simulink model "eVTOL_PX4_2023b"  (R2024b)
settings: Solver=ode4  StartTime=0  StopTime=inf  FixedStep=0.01  RelTol=1e-3
values from neighbouring files (symbols this model uses):
  aDl =     [initdata.mat]
  aDr =     [initdata.mat]
  aDyn =     [initdata.mat]
  Airport = init_airport('PHNL')    [initdata_HIL_eVTOL.m]
  aLat =     [initdata.mat]
  aLon =     [initdata.mat]
  D = Prop.D    [EOM_dt_MC.m]    (also in EOM_get_alf_dt_de_prop_evtol.m = CD * QS)
  dt0 = X(2)    [EOM_get_alf_dt_de_prop_evtol.m]    (also in initdata.mat = 0.258252593971; initdata_HIL_eVTOL.m = EOM_dt_MC)
  EAS0 = TAS0 / EAS2TAS    [initdata_HIL_eVTOL.m]
  FCS = init_FCS    [initdata_HIL_eVTOL.m]
  General = init_layoutdata    [EOM_dt_MC.m]    (also in build_optimized_CA.m; initdata.mat = ; initdata_HIL_eVTOL.m)
  h0 = Con(1)    [EOM_get_alf_dt_de_prop_evtol.m]    (also in initdata.mat = 450; initdata_HIL_eVTOL.m = 50)
  mass = Con(3)    [EOM_get_alf_dt_de_prop_evtol.m]    (also in initdata.mat = 2255.54; initdata_HIL_eVTOL.m = 7)
  Motor = init_motor_evtol    [EOM_dt_MC.m]    (also in initdata.mat = []; initdata_HIL_eVTOL.m)
  Prop = init_propeller_evtol_new    [EOM_dt_MC.m]    (also in initdata_HIL_eVTOL.m)
  R2D = 180/pi    (= 57.2957795131)    [EOM_get_alf_dt_de_prop_evtol.m]    (also in init_FCS.m; init_aerodata_evtol.m; init_airport.m; initdata.mat)
  SAMPLE_TIME = 0.01    [initdata_HIL_eVTOL.m]
  theta0 = -0.0510981441662    [initdata.mat]
undefined symbols (not defined in the file or in its folder): A1, aDa, aDe, aero, asbhl20env, B1, C1, de0, Earth, Environment, INIT_Data, InitData, Kd, Kp, magnitude, Newton, pProp, Raphson, Tc, WGS84
libraries: simulink_extras x63, vrlib x48, sharedtransform x28, simulink x22, slpidlib x20, sharedutil x20, matrix_library x18, aerolibwindfilters x12, aerolibobsolete x8, aerolibasang x8, aerolibatmos2 x6, aerolibfltsims x6
(part 5 of 17)

== system eVTOL_PX4_2023b/FCS/MC/att control1 ==
  DCM : Inport
  Att : Inport  Port=2
  Att_c : Inport  Port=3
  Add : Sum  Commented=on  Inputs=+++
  Att_c scp : Scope
  Demux1 : Demux  Outputs=3
  Demux2 : Demux  Outputs=3
  Derivative : Derivative  Commented=on
  Gain2 : Gain  Commented=on  Gain=0.5
  Gain3 : Gain  Gain=[0,0,1]
  Gain4 : Gain  Gain=[1,0,0]
  Gain6 : Gain  Gain=[0,1,0]
  Gain7 : Gain  Commented=on  Gain=0
  Gain8 : Gain  Commented=on  Gain=0
  Integrator : Integrator  Commented=on
  PID Controller : slpidlib/PID Controller  Controller=PID  Form=Parallel  TimeDomain=Continuous-time  UseExternalTs=off  SampleTime=-1  IntegratorMethod=Forward Euler  FilterMethod=Forward Euler  ControllerParametersSource=internal  P=2  I=0.5  UseKiTs=off  D=0.1  N=100  UseFilter=on  TunerSelectOption=Transfer Function Based (PID Tuner App)  InitialConditionSource=internal  InitialConditionForIntegrator=0  InitialConditionForFilter=0  DifferentiatorICPrevScaledInput=0  ExternalReset=none  TrackingMode=off  Kt=1  LimitOutput=on  SatLimitsSource=internal  UpperSaturationLimit=1.5  LowerSaturationLimit=-1.5  LinearizeAsGain=on  AntiWindupMode=clamping  Kb=1  LimitIntegrator=off  UpperIntegratorSaturationLimit=inf  LowerIntegratorSaturationLimit=-inf  POutMin=[]  POutMax=[]  IOutMin=[]  IOutMax=[]  DOutMin=[]  DOutMax=[]  NOutMin=[]  NOutMax=[]  SumOutMin=[]  SumOutMax=[]  SaturationOutMin=[]  SaturationOutMax=[]  PParamMin=[]  PParamMax=[]  IParamMin=[]  IParamMax=[]  DParamMin=[]  DParamMax=[]  NParamMin=[]  NParamMax=[]  KbParamMin=[]  KbParamMax=[]  KtParamMin=[]  KtParamMax=[]  KbOutMin=[]  KbOutMax=[]  KtOutMin=[]  KtOutMax=[]  IntegratorOutMin=[]  IntegratorOutMax=[]  FilterOutMin=[]  FilterOutMax=[]  SumI1OutMin=[]  SumI1OutMax=[]  SumI2OutMin=[]  SumI2OutMax=[]  SumI3OutMin=[]  SumI3OutMax=[]  SumI4OutMin=[]  SumI4OutMax=[]  SumDOutMin=[]  SumDOutMax=[]  DifferentiatorOutMin=[]  DifferentiatorOutMax=[]  FilterDiffOutCoefMin=[]  FilterDiffOutCoefMax=[]  ReciprocalOutMin=[]  ReciprocalOutMax=[]  SumDenOutMin=[]  SumDenOutMax=[]  SumNumOutMin=[]  SumNumOutMax=[]  DivideOutMin=[]  DivideOutMax=[]  UdiffTsProdOutMin=[]  UdiffTsProdOutMax=[]  NTsProdOutMin=[]  NTsProdOutMax=[]  UintegralTsProdOutMin=[]  UintegralTsProdOutMax=[]  UngainTsProdOutMin=[]  UngainTsProdOutMax=[]  ClampingZeroOutDataTypeStr=Inherit: Inherit via back propagation  ClampingZeroOutMin=[]  ClampingZeroOutMax=[]  FilterDenConstantOutDataTypeStr=Inherit: Inherit via back propagation  FilterDenConstantOutMin=[]  FilterDenConstantOutMax=[]  PCopyOutDataTypeStr=Inherit: Inherit via back propagation  PCopyOutMin=[]  PCopyOutMax=[]  NCopyOutDataTypeStr=Inherit: Inherit via back propagation  NCopyOutMin=[]  NCopyOutMax=[]  IntegratorContinuousStateAttributes=''  IntegratorStateMustResolveToSignalObject=off  IntegratorRTWStateStorageClass=Auto  FilterContinuousStateAttributes=''  FilterStateMustResolveToSignalObject=off  FilterRTWStateStorageClass=Auto  ParallelPVariant=InternalParameters  IdealPVariant=Disabled  IVariant=InternalParameters  DVariant=InternalParameters  IntegratorVariant=Continuous  SatVariant=Enabled  AWVariant=ContClampingParallel  PCopyVariant=Disabled  TRVariant=Disabled  FdbkBlocksVariant=Forward  IdealPFdbkVariant=Disabled  SatFdbkVariant=Disabled  DerivativeFilterVariant=ContFilter  NVariant=InternalParameters  NCopyVariant=Disabled  FilterICVariant=InternalICsFilter  IntegratorICVariant=InternalICs  ExternalResetVariant=Disabled  TRSumVariant=Passthrough  SumFdbkVariant=Disabled  SumVariant=Sum_PID  TsampFilterVariant=InternalTs  TsampNgainVariant=Passthrough  TsampIntegralVariant=Disabled_SignalSpec  ExternalSaturationOutDataTypeStr=Inherit: Same as second input
  PID Controller1 : slpidlib/PID Controller  Controller=PID  Form=Parallel  TimeDomain=Continuous-time  UseExternalTs=off  SampleTime=-1  IntegratorMethod=Forward Euler  FilterMethod=Forward Euler  ControllerParametersSource=internal  P=2  I=0.5  UseKiTs=off  D=0.1  N=100  UseFilter=on  TunerSelectOption=Transfer Function Based (PID Tuner App)  InitialConditionSource=internal  InitialConditionForIntegrator=0  InitialConditionForFilter=0  DifferentiatorICPrevScaledInput=0  ExternalReset=none  TrackingMode=off  Kt=1  LimitOutput=on  SatLimitsSource=internal  UpperSaturationLimit=1.5  LowerSaturationLimit=-1.5  LinearizeAsGain=on  AntiWindupMode=clamping  Kb=1  LimitIntegrator=off  UpperIntegratorSaturationLimit=inf  LowerIntegratorSaturationLimit=-inf  POutMin=[]  POutMax=[]  IOutMin=[]  IOutMax=[]  DOutMin=[]  DOutMax=[]  NOutMin=[]  NOutMax=[]  SumOutMin=[]  SumOutMax=[]  SaturationOutMin=[]  SaturationOutMax=[]  PParamMin=[]  PParamMax=[]  IParamMin=[]  IParamMax=[]  DParamMin=[]  DParamMax=[]  NParamMin=[]  NParamMax=[]  KbParamMin=[]  KbParamMax=[]  KtParamMin=[]  KtParamMax=[]  KbOutMin=[]  KbOutMax=[]  KtOutMin=[]  KtOutMax=[]  IntegratorOutMin=[]  IntegratorOutMax=[]  FilterOutMin=[]  FilterOutMax=[]  SumI1OutMin=[]  SumI1OutMax=[]  SumI2OutMin=[]  SumI2OutMax=[]  SumI3OutMin=[]  SumI3OutMax=[]  SumI4OutMin=[]  SumI4OutMax=[]  SumDOutMin=[]  SumDOutMax=[]  DifferentiatorOutMin=[]  DifferentiatorOutMax=[]  FilterDiffOutCoefMin=[]  FilterDiffOutCoefMax=[]  ReciprocalOutMin=[]  ReciprocalOutMax=[]  SumDenOutMin=[]  SumDenOutMax=[]  SumNumOutMin=[]  SumNumOutMax=[]  DivideOutMin=[]  DivideOutMax=[]  UdiffTsProdOutMin=[]  UdiffTsProdOutMax=[]  NTsProdOutMin=[]  NTsProdOutMax=[]  UintegralTsProdOutMin=[]  UintegralTsProdOutMax=[]  UngainTsProdOutMin=[]  UngainTsProdOutMax=[]  ClampingZeroOutDataTypeStr=Inherit: Inherit via back propagation  ClampingZeroOutMin=[]  ClampingZeroOutMax=[]  FilterDenConstantOutDataTypeStr=Inherit: Inherit via back propagation  FilterDenConstantOutMin=[]  FilterDenConstantOutMax=[]  PCopyOutDataTypeStr=Inherit: Inherit via back propagation  PCopyOutMin=[]  PCopyOutMax=[]  NCopyOutDataTypeStr=Inherit: Inherit via back propagation  NCopyOutMin=[]  NCopyOutMax=[]  IntegratorContinuousStateAttributes=''  IntegratorStateMustResolveToSignalObject=off  IntegratorRTWStateStorageClass=Auto  FilterContinuousStateAttributes=''  FilterStateMustResolveToSignalObject=off  FilterRTWStateStorageClass=Auto  ParallelPVariant=InternalParameters  IdealPVariant=Disabled  IVariant=InternalParameters  DVariant=InternalParameters  IntegratorVariant=Continuous  SatVariant=Enabled  AWVariant=ContClampingParallel  PCopyVariant=Disabled  TRVariant=Disabled  FdbkBlocksVariant=Forward  IdealPFdbkVariant=Disabled  SatFdbkVariant=Disabled  DerivativeFilterVariant=ContFilter  NVariant=InternalParameters  NCopyVariant=Disabled  FilterICVariant=InternalICsFilter  IntegratorICVariant=InternalICs  ExternalResetVariant=Disabled  TRSumVariant=Passthrough  SumFdbkVariant=Disabled  SumVariant=Sum_PID  TsampFilterVariant=InternalTs  TsampNgainVariant=Passthrough  TsampIntegralVariant=Disabled_SignalSpec  ExternalSaturationOutDataTypeStr=Inherit: Same as second input
  PID Controller2 : slpidlib/PID Controller  Controller=PI  Form=Parallel  TimeDomain=Continuous-time  UseExternalTs=off  SampleTime=-1  IntegratorMethod=Forward Euler  FilterMethod=Forward Euler  ControllerParametersSource=internal  P=2  I=0.5  UseKiTs=off  D=0  N=100  UseFilter=on  TunerSelectOption=Transfer Function Based (PID Tuner App)  InitialConditionSource=internal  InitialConditionForIntegrator=0  InitialConditionForFilter=0  DifferentiatorICPrevScaledInput=0  ExternalReset=none  TrackingMode=off  Kt=1  LimitOutput=on  SatLimitsSource=internal  UpperSaturationLimit=25/57.3  LowerSaturationLimit=-25/57.3  LinearizeAsGain=on  AntiWindupMode=none  Kb=1  LimitIntegrator=off  UpperIntegratorSaturationLimit=inf  LowerIntegratorSaturationLimit=-inf  POutMin=[]  POutMax=[]  IOutMin=[]  IOutMax=[]  DOutMin=[]  DOutMax=[]  NOutMin=[]  NOutMax=[]  SumOutMin=[]  SumOutMax=[]  SaturationOutMin=[]  SaturationOutMax=[]  PParamMin=[]  PParamMax=[]  IParamMin=[]  IParamMax=[]  DParamMin=[]  DParamMax=[]  NParamMin=[]  NParamMax=[]  KbParamMin=[]  KbParamMax=[]  KtParamMin=[]  KtParamMax=[]  KbOutMin=[]  KbOutMax=[]  KtOutMin=[]  KtOutMax=[]  IntegratorOutMin=[]  IntegratorOutMax=[]  FilterOutMin=[]  FilterOutMax=[]  SumI1OutMin=[]  SumI1OutMax=[]  SumI2OutMin=[]  SumI2OutMax=[]  SumI3OutMin=[]  SumI3OutMax=[]  SumI4OutMin=[]  SumI4OutMax=[]  SumDOutMin=[]  SumDOutMax=[]  DifferentiatorOutMin=[]  DifferentiatorOutMax=[]  FilterDiffOutCoefMin=[]  FilterDiffOutCoefMax=[]  ReciprocalOutMin=[]  ReciprocalOutMax=[]  SumDenOutMin=[]  SumDenOutMax=[]  SumNumOutMin=[]  SumNumOutMax=[]  DivideOutMin=[]  DivideOutMax=[]  UdiffTsProdOutMin=[]  UdiffTsProdOutMax=[]  NTsProdOutMin=[]  NTsProdOutMax=[]  UintegralTsProdOutMin=[]  UintegralTsProdOutMax=[]  UngainTsProdOutMin=[]  UngainTsProdOutMax=[]  ClampingZeroOutDataTypeStr=Inherit: Inherit via back propagation  ClampingZeroOutMin=[]  ClampingZeroOutMax=[]  FilterDenConstantOutDataTypeStr=Inherit: Inherit via back propagation  FilterDenConstantOutMin=[]  FilterDenConstantOutMax=[]  PCopyOutDataTypeStr=Inherit: Inherit via back propagation  PCopyOutMin=[]  PCopyOutMax=[]  NCopyOutDataTypeStr=Inherit: Inherit via back propagation  NCopyOutMin=[]  NCopyOutMax=[]  IntegratorContinuousStateAttributes=''  IntegratorStateMustResolveToSignalObject=off  IntegratorRTWStateStorageClass=Auto  FilterContinuousStateAttributes=''  FilterStateMustResolveToSignalObject=off  FilterRTWStateStorageClass=Auto  ParallelPVariant=InternalParameters  IdealPVariant=Disabled  IVariant=InternalParameters  DVariant=Disabled  IntegratorVariant=Continuous  SatVariant=Enabled  AWVariant=Passthrough  PCopyVariant=Disabled  TRVariant=Disabled  FdbkBlocksVariant=Forward  IdealPFdbkVariant=Disabled  SatFdbkVariant=Disabled  DerivativeFilterVariant=Disabled  NVariant=Disabled  NCopyVariant=Disabled_SignalSpec  FilterICVariant=Disabled  IntegratorICVariant=InternalICs  ExternalResetVariant=Disabled  TRSumVariant=Passthrough  SumFdbkVariant=Disabled  SumVariant=Sum_PI  TsampFilterVariant=InternalTs  TsampNgainVariant=Passthrough  TsampIntegralVariant=Disabled_SignalSpec  ExternalSaturationOutDataTypeStr=Inherit: Same as second input
  Product1 : Product  Multiplication=Matrix(*)
  Radians to Degrees1 : simulink_extras/Transformations/Radians to Degrees
  Radians to Degrees2 : simulink_extras/Transformations/Radians to Degrees
  Radians to Degrees3 : simulink_extras/Transformations/Radians to Degrees
  Scope : Scope  NumInputPorts=2
  Scope1 : Scope  NumInputPorts=2
  Scope2 : Scope  NumInputPorts=2
  Sine Wave : Sin  SampleTime=0
  Sum3 : Sum  Inputs=|+-
  Sum5 : Sum  Inputs=|+-
  Sum7 : Sum  Inputs=|+-
  Sum8 : Sum  Inputs=+++
  pqr_c : Outport
  wires:
  Gain4/1 -> Sum8/1  "pc"
  Demux1/2 -> [theta]
  Sum3/1 -> PID Controller1/1
  [phi] -> Sum3/2, Scope1/2  "phi"
  [psi] -> Radians to Degrees3/1, Sum5/2
  Gain6/1 -> Sum8/2  "qc"
  [psi_c] -> Radians to Degrees2/1, Sum5/1
  Att/1 -> Demux1/1
  Sum7/1 -> PID Controller/1
  Sum8/1 -> Product1/2
  PID Controller1/1 -> Gain4/1  "phi_dot_c"
  Demux1/3 -> [psi]
  Gain2/1 -> Add/2
  Gain3/1 -> Sum8/3  "rc"
  Demux1/1 -> [phi]
  DCM/1 -> Product1/1
  Product1/1 -> pqr_c/1
  Demux2/1 -> [phi_c]
  Demux2/2 -> [theta_c]
  Demux2/3 -> [psi_c]
  Att_c/1 -> Radians to Degrees1/1, Demux2/1
  [phi_c] -> Scope1/1, Sum3/1  "phi_c"
  Radians to Degrees1/1 -> Att_c scp/1
  Radians to Degrees2/1 -> Scope/1
  Radians to Degrees3/1 -> Scope/2
  PID Controller/1 -> Gain6/1
  [theta] -> Scope2/2, Sum7/2  "theta"
  Gain7/1 -> Add/3
  Derivative/1 -> Gain7/1
  Integrator/1 -> Gain8/1
  Gain8/1 -> Add/1
  [theta_c] -> Scope2/1, Sum7/1  "theta_c"
  Sum5/1 -> PID Controller2/1
  PID Controller2/1 -> Gain3/1

== system eVTOL_PX4_2023b/FCS/MC/rate control ==
  note: [pc,rc]_b = rc_e*[-1,1]
      | [pc,rc]_b = pc_e*[1,1]
  pqr : Inport
  pqr_c : Inport  Port=2
  Demux5 : Demux  Outputs=3
  Demux6 : Demux  Outputs=3
  PID Controller : slpidlib/PID Controller  Controller=PID  Form=Parallel  TimeDomain=Continuous-time  UseExternalTs=off  SampleTime=-1  IntegratorMethod=Forward Euler  FilterMethod=Forward Euler  ControllerParametersSource=internal  P=1.5  I=0.2  UseKiTs=off  D=0.35  N=36.3717094270686  UseFilter=on  TunerSelectOption=Transfer Function Based (PID Tuner App)  InitialConditionSource=internal  InitialConditionForIntegrator=0  InitialConditionForFilter=0  DifferentiatorICPrevScaledInput=0  ExternalReset=none  TrackingMode=off  Kt=1  LimitOutput=on  SatLimitsSource=internal  UpperSaturationLimit=0.6  LowerSaturationLimit=-0.6  LinearizeAsGain=on  AntiWindupMode=clamping  Kb=1  LimitIntegrator=off  UpperIntegratorSaturationLimit=inf  LowerIntegratorSaturationLimit=-inf  POutMin=[]  POutMax=[]  IOutMin=[]  IOutMax=[]  DOutMin=[]  DOutMax=[]  NOutMin=[]  NOutMax=[]  SumOutMin=[]  SumOutMax=[]  SaturationOutMin=[]  SaturationOutMax=[]  PParamMin=[]  PParamMax=[]  IParamMin=[]  IParamMax=[]  DParamMin=[]  DParamMax=[]  NParamMin=[]  NParamMax=[]  KbParamMin=[]  KbParamMax=[]  KtParamMin=[]  KtParamMax=[]  KbOutMin=[]  KbOutMax=[]  KtOutMin=[]  KtOutMax=[]  IntegratorOutMin=[]  IntegratorOutMax=[]  FilterOutMin=[]  FilterOutMax=[]  SumI1OutMin=[]  SumI1OutMax=[]  SumI2OutMin=[]  SumI2OutMax=[]  SumI3OutMin=[]  SumI3OutMax=[]  SumI4OutMin=[]  SumI4OutMax=[]  SumDOutMin=[]  SumDOutMax=[]  DifferentiatorOutMin=[]  DifferentiatorOutMax=[]  FilterDiffOutCoefMin=[]  FilterDiffOutCoefMax=[]  ReciprocalOutMin=[]  ReciprocalOutMax=[]  SumDenOutMin=[]  SumDenOutMax=[]  SumNumOutMin=[]  SumNumOutMax=[]  DivideOutMin=[]  DivideOutMax=[]  UdiffTsProdOutMin=[]  UdiffTsProdOutMax=[]  NTsProdOutMin=[]  NTsProdOutMax=[]  UintegralTsProdOutMin=[]  UintegralTsProdOutMax=[]  UngainTsProdOutMin=[]  UngainTsProdOutMax=[]  ClampingZeroOutDataTypeStr=Inherit: Inherit via back propagation  ClampingZeroOutMin=[]  ClampingZeroOutMax=[]  FilterDenConstantOutDataTypeStr=Inherit: Inherit via back propagation  FilterDenConstantOutMin=[]  FilterDenConstantOutMax=[]  PCopyOutDataTypeStr=Inherit: Inherit via back propagation  PCopyOutMin=[]  PCopyOutMax=[]  NCopyOutDataTypeStr=Inherit: Inherit via back propagation  NCopyOutMin=[]  NCopyOutMax=[]  IntegratorContinuousStateAttributes=''  IntegratorStateMustResolveToSignalObject=off  IntegratorRTWStateStorageClass=Auto  FilterContinuousStateAttributes=''  FilterStateMustResolveToSignalObject=off  FilterRTWStateStorageClass=Auto  ParallelPVariant=InternalParameters  IdealPVariant=Disabled  IVariant=InternalParameters  DVariant=InternalParameters  IntegratorVariant=Continuous  SatVariant=Enabled  AWVariant=ContClampingParallel  PCopyVariant=Disabled  TRVariant=Disabled  FdbkBlocksVariant=Forward  IdealPFdbkVariant=Disabled  SatFdbkVariant=Disabled  DerivativeFilterVariant=ContFilter  NVariant=InternalParameters  NCopyVariant=Disabled  FilterICVariant=InternalICsFilter  IntegratorICVariant=InternalICs  ExternalResetVariant=Disabled  TRSumVariant=Passthrough  SumFdbkVariant=Disabled  SumVariant=Sum_PID  TsampFilterVariant=InternalTs  TsampNgainVariant=Passthrough  TsampIntegralVariant=Disabled_SignalSpec  ExternalSaturationOutDataTypeStr=Inherit: Same as second input
  PID Controller2 : slpidlib/PID Controller  Controller=PID  Form=Parallel  TimeDomain=Continuous-time  UseExternalTs=off  SampleTime=-1  IntegratorMethod=Forward Euler  FilterMethod=Forward Euler  ControllerParametersSource=internal  P=25  I=3.5  UseKiTs=off  D=6  N=39.8807863432362  UseFilter=on  TunerSelectOption=Transfer Function Based (PID Tuner App)  InitialConditionSource=internal  InitialConditionForIntegrator=0  InitialConditionForFilter=0  DifferentiatorICPrevScaledInput=0  ExternalReset=none  TrackingMode=off  Kt=1  LimitOutput=on  SatLimitsSource=internal  UpperSaturationLimit=1.2  LowerSaturationLimit=-1.2  LinearizeAsGain=on  AntiWindupMode=clamping  Kb=1  LimitIntegrator=off  UpperIntegratorSaturationLimit=inf  LowerIntegratorSaturationLimit=-inf  POutMin=[]  POutMax=[]  IOutMin=[]  IOutMax=[]  DOutMin=[]  DOutMax=[]  NOutMin=[]  NOutMax=[]  SumOutMin=[]  SumOutMax=[]  SaturationOutMin=[]  SaturationOutMax=[]  PParamMin=[]  PParamMax=[]  IParamMin=[]  IParamMax=[]  DParamMin=[]  DParamMax=[]  NParamMin=[]  NParamMax=[]  KbParamMin=[]  KbParamMax=[]  KtParamMin=[]  KtParamMax=[]  KbOutMin=[]  KbOutMax=[]  KtOutMin=[]  KtOutMax=[]  IntegratorOutMin=[]  IntegratorOutMax=[]  FilterOutMin=[]  FilterOutMax=[]  SumI1OutMin=[]  SumI1OutMax=[]  SumI2OutMin=[]  SumI2OutMax=[]  SumI3OutMin=[]  SumI3OutMax=[]  SumI4OutMin=[]  SumI4OutMax=[]  SumDOutMin=[]  SumDOutMax=[]  DifferentiatorOutMin=[]  DifferentiatorOutMax=[]  FilterDiffOutCoefMin=[]  FilterDiffOutCoefMax=[]  ReciprocalOutMin=[]  ReciprocalOutMax=[]  SumDenOutMin=[]  SumDenOutMax=[]  SumNumOutMin=[]  SumNumOutMax=[]  DivideOutMin=[]  DivideOutMax=[]  UdiffTsProdOutMin=[]  UdiffTsProdOutMax=[]  NTsProdOutMin=[]  NTsProdOutMax=[]  UintegralTsProdOutMin=[]  UintegralTsProdOutMax=[]  UngainTsProdOutMin=[]  UngainTsProdOutMax=[]  ClampingZeroOutDataTypeStr=Inherit: Inherit via back propagation  ClampingZeroOutMin=[]  ClampingZeroOutMax=[]  FilterDenConstantOutDataTypeStr=Inherit: Inherit via back propagation  FilterDenConstantOutMin=[]  FilterDenConstantOutMax=[]  PCopyOutDataTypeStr=Inherit: Inherit via back propagation  PCopyOutMin=[]  PCopyOutMax=[]  NCopyOutDataTypeStr=Inherit: Inherit via back propagation  NCopyOutMin=[]  NCopyOutMax=[]  IntegratorContinuousStateAttributes=''  IntegratorStateMustResolveToSignalObject=off  IntegratorRTWStateStorageClass=Auto  FilterContinuousStateAttributes=''  FilterStateMustResolveToSignalObject=off  FilterRTWStateStorageClass=Auto  ParallelPVariant=InternalParameters  IdealPVariant=Disabled  IVariant=InternalParameters  DVariant=InternalParameters  IntegratorVariant=Continuous  SatVariant=Enabled  AWVariant=ContClampingParallel  PCopyVariant=Disabled  TRVariant=Disabled  FdbkBlocksVariant=Forward  IdealPFdbkVariant=Disabled  SatFdbkVariant=Disabled  DerivativeFilterVariant=ContFilter  NVariant=InternalParameters  NCopyVariant=Disabled  FilterICVariant=InternalICsFilter  IntegratorICVariant=InternalICs  ExternalResetVariant=Disabled  TRSumVariant=Passthrough  SumFdbkVariant=Disabled  SumVariant=Sum_PID  TsampFilterVariant=InternalTs  TsampNgainVariant=Passthrough  TsampIntegralVariant=Disabled_SignalSpec  ExternalSaturationOutDataTypeStr=Inherit: Same as second input
  PID Controller3 : slpidlib/PID Controller  Controller=PID  Form=Parallel  TimeDomain=Continuous-time  UseExternalTs=off  SampleTime=-1  IntegratorMethod=Forward Euler  FilterMethod=Forward Euler  ControllerParametersSource=internal  P=3.3837424696878  I=2.17144539151316  UseKiTs=off  D=1.038917423344  N=48.7666926128464  UseFilter=on  TunerSelectOption=Transfer Function Based (PID Tuner App)  InitialConditionSource=internal  InitialConditionForIntegrator=0  InitialConditionForFilter=0  DifferentiatorICPrevScaledInput=0  ExternalReset=none  TrackingMode=off  Kt=1  LimitOutput=on  SatLimitsSource=internal  UpperSaturationLimit=0.8  LowerSaturationLimit=-0.8  LinearizeAsGain=on  AntiWindupMode=clamping  Kb=1  LimitIntegrator=off  UpperIntegratorSaturationLimit=inf  LowerIntegratorSaturationLimit=-inf  POutMin=[]  POutMax=[]  IOutMin=[]  IOutMax=[]  DOutMin=[]  DOutMax=[]  NOutMin=[]  NOutMax=[]  SumOutMin=[]  SumOutMax=[]  SaturationOutMin=[]  SaturationOutMax=[]  PParamMin=[]  PParamMax=[]  IParamMin=[]  IParamMax=[]  DParamMin=[]  DParamMax=[]  NParamMin=[]  NParamMax=[]  KbParamMin=[]  KbParamMax=[]  KtParamMin=[]  KtParamMax=[]  KbOutMin=[]  KbOutMax=[]  KtOutMin=[]  KtOutMax=[]  IntegratorOutMin=[]  IntegratorOutMax=[]  FilterOutMin=[]  FilterOutMax=[]  SumI1OutMin=[]  SumI1OutMax=[]  SumI2OutMin=[]  SumI2OutMax=[]  SumI3OutMin=[]  SumI3OutMax=[]  SumI4OutMin=[]  SumI4OutMax=[]  SumDOutMin=[]  SumDOutMax=[]  DifferentiatorOutMin=[]  DifferentiatorOutMax=[]  FilterDiffOutCoefMin=[]  FilterDiffOutCoefMax=[]  ReciprocalOutMin=[]  ReciprocalOutMax=[]  SumDenOutMin=[]  SumDenOutMax=[]  SumNumOutMin=[]  SumNumOutMax=[]  DivideOutMin=[]  DivideOutMax=[]  UdiffTsProdOutMin=[]  UdiffTsProdOutMax=[]  NTsProdOutMin=[]  NTsProdOutMax=[]  UintegralTsProdOutMin=[]  UintegralTsProdOutMax=[]  UngainTsProdOutMin=[]  UngainTsProdOutMax=[]  ClampingZeroOutDataTypeStr=Inherit: Inherit via back propagation  ClampingZeroOutMin=[]  ClampingZeroOutMax=[]  FilterDenConstantOutDataTypeStr=Inherit: Inherit via back propagation  FilterDenConstantOutMin=[]  FilterDenConstantOutMax=[]  PCopyOutDataTypeStr=Inherit: Inherit via back propagation  PCopyOutMin=[]  PCopyOutMax=[]  NCopyOutDataTypeStr=Inherit: Inherit via back propagation  NCopyOutMin=[]  NCopyOutMax=[]  IntegratorContinuousStateAttributes=''  IntegratorStateMustResolveToSignalObject=off  IntegratorRTWStateStorageClass=Auto  FilterContinuousStateAttributes=''  FilterStateMustResolveToSignalObject=off  FilterRTWStateStorageClass=Auto  ParallelPVariant=InternalParameters  IdealPVariant=Disabled  IVariant=InternalParameters  DVariant=InternalParameters  IntegratorVariant=Continuous  SatVariant=Enabled  AWVariant=ContClampingParallel  PCopyVariant=Disabled  TRVariant=Disabled  FdbkBlocksVariant=Forward  IdealPFdbkVariant=Disabled  SatFdbkVariant=Disabled  DerivativeFilterVariant=ContFilter  NVariant=InternalParameters  NCopyVariant=Disabled  FilterICVariant=InternalICsFilter  IntegratorICVariant=InternalICs  ExternalResetVariant=Disabled  TRSumVariant=Passthrough  SumFdbkVariant=Disabled  SumVariant=Sum_PID  TsampFilterVariant=InternalTs  TsampNgainVariant=Passthrough  TsampIntegralVariant=Disabled_SignalSpec  ExternalSaturationOutDataTypeStr=Inherit: Same as second input
  Radians to Degrees : simulink_extras/Transformations/Radians to Degrees
  Radians to Degrees1 : simulink_extras/Transformations/Radians to Degrees
  Saturation : Saturate  UpperLimit=30/57.3  LowerLimit=-30/57.3
  Saturation1 : Saturate  UpperLimit=0.2  LowerLimit=-0.2
  Saturation2 : Saturate  UpperLimit=0.2  LowerLimit=-0.2
  Scope : Scope  NumInputPorts=2
  Scope1 : Scope  NumInputPorts=2
  Scope2 : Scope  NumInputPorts=2
  Sum : Sum  Inputs=|+-
  Sum2 : Sum  Inputs=|+-
  Sum4 : Sum  Inputs=|+-
  pqr scp : Scope
  pqr_c scp : Scope
  da_MC : Outport
  de_MC : Outport  Port=2
  dr_MC : Outport  Port=3
  wires:
  [qc] -> Saturation2/1  "qc"
  [q] -> Sum/2, Scope/2  "q"
  [p] -> Scope2/1, Sum2/2
  PID Controller3/1 -> de_MC/1
  [r] -> Scope1/2, Sum4/2  "r"
  Sum4/1 -> PID Controller2/1
  Sum2/1 -> PID Controller/1
  [rc] -> Saturation/1  "rc"
  [pc] -> Saturation1/1  "pc"
  PID Controller/1 -> da_MC/1
  Demux5/1 -> [p]
  Demux5/2 -> [q]
  Demux5/3 -> [r]
  pqr_c/1 -> Radians to Degrees/1, Demux6/1
  Demux6/3 -> [rc]
  Demux6/1 -> [pc]
  Demux6/2 -> [qc]
  Saturation1/1 -> Scope2/2, Sum2/1
  pqr/1 -> Radians to Degrees1/1, Demux5/1
  PID Controller2/1 -> dr_MC/1
  Radians to Degrees/1 -> pqr_c scp/1
  Radians to Degrees1/1 -> pqr scp/1
  Sum/1 -> PID Controller3/1
  Saturation2/1 -> Scope/1, Sum/1  "qc"
  Saturation/1 -> Scope1/1, Sum4/1

== system eVTOL_PX4_2023b/FCS/control selector/Switch Case Action Subsystem1 ==
  In1 : Inport
  Action Port : ActionPort
  Out1 : Outport  VectorParamsAs1DForOutWhenUnconnected=off
  wires:
  In1/1 -> Out1/1

== system eVTOL_PX4_2023b/FCS/control selector/Switch Case Action Subsystem2 ==
  In1 : Inport
  Action Port : ActionPort
  Out1 : Outport  VectorParamsAs1DForOutWhenUnconnected=off
  wires:
  In1/1 -> Out1/1

== system eVTOL_PX4_2023b/Subsystem1/Energy & Power/V_prop1 ==
  note: 将速度矢量投影到桨轴
  pqr : Inport
  pos : Inport  Port=2
  i : Inport  Port=3
  Vb : Inport  Port=4
  Cross Product4 : matrix_library/Cross Product
  Display1 : Display
  Display2 : Display
  Display8 : Display
  Sum2 : Sum  Inputs=|++
  v_b to v_prop : Subsystem
  V : Outport
  wires:
  pos/1 -> Cross Product4/2
  pqr/1 -> Cross Product4/1
  Vb/1 -> Display2/1, Sum2/2
  i/1 -> v_b to v_prop/2(i)
  Cross Product4/1 -> Display8/1, Sum2/1
  Sum2/1 -> Display1/1, v_b to v_prop/1(V_body)
  v_b to v_prop/1(V) -> V/1

== system eVTOL_PX4_2023b/Subsystem1/Energy & Power/V_prop2 ==
  note: 将速度矢量投影到桨轴
  pqr : Inport
  pos : Inport  Port=2
  i : Inport  Port=3
  Vb : Inport  Port=4
  Cross Product4 : matrix_library/Cross Product
  Sum2 : Sum  Inputs=|++
  v_b to v_prop : Subsystem
  V : Outport
  wires:
  pos/1 -> Cross Product4/2
  pqr/1 -> Cross Product4/1
  Vb/1 -> Sum2/2
  i/1 -> v_b to v_prop/2(i)
  Cross Product4/1 -> Sum2/1
  Sum2/1 -> v_b to v_prop/1(V_body)
  v_b to v_prop/1(V) -> V/1

== system eVTOL_PX4_2023b/Subsystem1/Energy & Power/V_prop3 ==
  note: 将速度矢量投影到桨轴
  pqr : Inport
  pos : Inport  Port=2
  i : Inport  Port=3
  Va : Inport  Port=4
  Cross Product4 : matrix_library/Cross Product
  Sum2 : Sum  Inputs=|++
  v_b to v_prop : Subsystem
  V : Outport
  wires:
  pos/1 -> Cross Product4/2
  pqr/1 -> Cross Product4/1
  Va/1 -> Sum2/2
  i/1 -> v_b to v_prop/2(i)
  Cross Product4/1 -> Sum2/1
  Sum2/1 -> v_b to v_prop/1(V_body)
  v_b to v_prop/1(V) -> V/1

== system eVTOL_PX4_2023b/Subsystem1/Energy & Power/V_prop4 ==
  note: 将速度矢量投影到桨轴
  pqr : Inport
  pos : Inport  Port=2
  i : Inport  Port=3
  Va : Inport  Port=4
  Cross Product4 : matrix_library/Cross Product
  Sum2 : Sum  Inputs=|++
  v_b to v_prop : Subsystem
  V : Outport
  wires:
  pos/1 -> Cross Product4/2
  pqr/1 -> Cross Product4/1
  Va/1 -> Sum2/2
  i/1 -> v_b to v_prop/2(i)
  Cross Product4/1 -> Sum2/1
  Sum2/1 -> v_b to v_prop/1(V_body)
  v_b to v_prop/1(V) -> V/1

== system eVTOL_PX4_2023b/Subsystem1/Energy & Power/V_prop5 ==
  note: 将速度矢量投影到桨轴
  pqr : Inport
  pos : Inport  Port=2
  i : Inport  Port=3
  Va : Inport  Port=4
  Cross Product4 : matrix_library/Cross Product
  Sum2 : Sum  Inputs=|++
  v_b to v_prop : Subsystem
  V : Outport
  wires:
  pos/1 -> Cross Product4/2
  pqr/1 -> Cross Product4/1
  Va/1 -> Sum2/2
  i/1 -> v_b to v_prop/2(i)
  Cross Product4/1 -> Sum2/1
  Sum2/1 -> v_b to v_prop/1(V_body)
  v_b to v_prop/1(V) -> V/1

== system eVTOL_PX4_2023b/Subsystem1/Energy & Power/V_prop6 ==
  note: 将速度矢量投影到桨轴
  pqr : Inport
  pos : Inport  Port=2
  i : Inport  Port=3
  Va : Inport  Port=4
  Cross Product4 : matrix_library/Cross Product
  Sum2 : Sum  Inputs=|++
  v_b to v_prop : Subsystem
  V : Outport
  wires:
  pos/1 -> Cross Product4/2
  pqr/1 -> Cross Product4/1
  Va/1 -> Sum2/2
  i/1 -> v_b to v_prop/2(i)
  Cross Product4/1 -> Sum2/1
  Sum2/1 -> v_b to v_prop/1(V_body)
  v_b to v_prop/1(V) -> V/1

== system eVTOL_PX4_2023b/Subsystem1/Energy & Power/thrust_1 ==
  note: 将推力、扭矩按电机倾转角转化为向量
  note: 求桨的推力、扭矩、功率、效率
  dt : Inport
  V : Inport  Port=2
  rho : Inport  Port=3
  rpm0 : Inport  Port=4
  theta_b : Inport  Port=5
  i : Inport  Port=6
  Constant : Constant  Commented=on  Value=2.5
  Gain2 : Gain  Gain=-1
  Gain4 : Gain  Gain=pi/30
  Manual Switch : ManualSwitch  Commented=on  CurrentSetting=0
  Motor : Subsystem
  Mux1 : Mux  Inputs=2
  Mux2 : Mux  Inputs=3
  Mux3 : Mux  Inputs=2
  Mux4 : Mux  Inputs=3
  Product : Product  Inputs=*/
  "Propeller " : Subsystem
  Q_x : Fcn  Expr=-u[1]*cos(u[2])
  Q_y : Fcn  Expr=0
  Q_z : Fcn  Expr=u[1]*sin(u[2])
  Saturation : Saturate  UpperLimit=inf  LowerLimit=1
  T_x : Fcn  Expr=u[1]*cos(u[2])
  T_y : Fcn  Expr=0
  T_z : Fcn  Expr=-u[1]*sin(u[2])
  eta_plr : Outport  VectorParamsAs1DForOutWhenUnconnected=off
  Q : Outport  Port=2
  T : Outport  Port=3  VectorParamsAs1DForOutWhenUnconnected=off
  rpm : Outport  Port=4  VectorParamsAs1DForOutWhenUnconnected=off
  wires:
  Saturation/1 -> Motor/4(rpm0)
  rpm0/1 -> Saturation/1
  "Propeller "/2(T (N)) -> [T]
  dt/1 -> Motor/2(dt)
  Motor/1(rpm) -> rpm/1, Gain4/1, "Propeller "/1(rpm)
  "Propeller "/3(eta_p) -> eta_plr/1
  rho/1 -> [rho]
  "Propeller "/1(P_plr (w)) -> Motor/1(P_shaft), Product/1
  theta_b/1 -> Motor/6(theta_b), "Propeller "/4(theta_b)
  Gain4/1 -> Product/2  "omega"
  Product/1 -> Gain2/1
  T_y/1 -> Mux2/2
  Mux1/1 -> T_z/1, T_x/1, T_y/1
  T_x/1 -> Mux2/1
  i/1 -> [i]
  T_z/1 -> Mux2/3
  Mux2/1 -> T/1
  [T] -> Mux1/1
  Mux4/1 -> Q/1
  [i] -> Mux3/2
  Q_z/1 -> Mux4/3
  Q_x/1 -> Mux4/1
  Mux3/1 -> Q_z/1, Q_x/1, Q_y/1
  Q_y/1 -> Mux4/2
  [Q] -> Mux3/1
  [i] -> Mux1/2
  Gain2/1 -> [Q]
  [V] -> Motor/3(V)
  [V] -> "Propeller "/2(V)
  [rho] -> Motor/5(rho)
  [rho] -> "Propeller "/3(rho)
  Constant/1 -> Manual Switch/1
  V/1 -> [V]

== system eVTOL_PX4_2023b/Subsystem1/Energy & Power/thrust_2 ==
  note: 将推力、扭矩按电机倾转角转化为向量
  note: 求桨的推力、扭矩、功率、效率
  dt : Inport
  V : Inport  Port=2
  rho : Inport  Port=3
  rpm0 : Inport  Port=4
  theta_b : Inport  Port=5
  i : Inport  Port=6
  Constant : Constant  Commented=on  Value=2.5
  Gain4 : Gain  Gain=pi/30
  Manual Switch : ManualSwitch  Commented=on  CurrentSetting=0
  Motor : Subsystem
  Mux1 : Mux  Inputs=2
  Mux2 : Mux  Inputs=3
  Mux3 : Mux  Inputs=2
  Mux4 : Mux  Inputs=3
  Product : Product  Inputs=*/
  "Propeller " : Subsystem
  Q_x : Fcn  Expr=-u[1]*cos(u[2])
  Q_y : Fcn  Expr=0
  Q_z : Fcn  Expr=u[1]*sin(u[2])
  Saturation : Saturate  UpperLimit=inf  LowerLimit=1
  T_x : Fcn  Expr=u[1]*cos(u[2])
  T_y : Fcn  Expr=0
  T_z : Fcn  Expr=-u[1]*sin(u[2])
  eta_plr : Outport  VectorParamsAs1DForOutWhenUnconnected=off
  Q : Outport  Port=2
  T : Outport  Port=3  VectorParamsAs1DForOutWhenUnconnected=off
  rpm : Outport  Port=4  VectorParamsAs1DForOutWhenUnconnected=off
  wires:
  Saturation/1 -> Motor/4(rpm0)
  rpm0/1 -> Saturation/1
  "Propeller "/2(T (N)) -> [T]
  dt/1 -> Motor/2(dt)
  Motor/1(rpm) -> rpm/1, Gain4/1, "Propeller "/1(rpm)
  "Propeller "/3(eta_p) -> eta_plr/1
  rho/1 -> [rho]
  "Propeller "/1(P_plr (w)) -> Motor/1(P_shaft), Product/1
  theta_b/1 -> Motor/6(theta_b), "Propeller "/4(theta_b)
  Gain4/1 -> Product/2  "omega"
  T_y/1 -> Mux2/2
  Mux1/1 -> T_z/1, T_x/1, T_y/1
  T_x/1 -> Mux2/1
  i/1 -> [i]
  T_z/1 -> Mux2/3
  Mux2/1 -> T/1
  [T] -> Mux1/1
  Mux4/1 -> Q/1
  [i] -> Mux3/2
  Q_z/1 -> Mux4/3
  Q_x/1 -> Mux4/1
  Mux3/1 -> Q_z/1, Q_x/1, Q_y/1
  Q_y/1 -> Mux4/2
  [Q] -> Mux3/1
  [i] -> Mux1/2
  Product/1 -> [Q]
  [V] -> Motor/3(V)
  [V] -> "Propeller "/2(V)
  [rho] -> Motor/5(rho)
  [rho] -> "Propeller "/3(rho)
  Constant/1 -> Manual Switch/1
  V/1 -> [V]

== system eVTOL_PX4_2023b/Subsystem1/Energy & Power/thrust_3 ==
  note: 将推力、扭矩按电机倾转角转化为向量
  note: 求桨的推力、扭矩、功率、效率
  dt : Inport
  V : Inport  Port=2
  rho : Inport  Port=3
  rpm0 : Inport  Port=4
  theta_b : Inport  Port=5
  i : Inport  Port=6
  Constant : Constant  Commented=on  Value=2.5
  Gain2 : Gain  Gain=-1
  Gain4 : Gain  Gain=pi/30
  Manual Switch : ManualSwitch  Commented=on  CurrentSetting=0
  Motor : Subsystem
  Mux1 : Mux  Inputs=2
  Mux2 : Mux  Inputs=3
  Mux3 : Mux  Inputs=2
  Mux4 : Mux  Inputs=3
  Product : Product  Inputs=*/
  "Propeller " : Subsystem
  Q_x : Fcn  Expr=-u[1]*cos(u[2])
  Q_y : Fcn  Expr=0
  Q_z : Fcn  Expr=u[1]*sin(u[2])
  Saturation : Saturate  UpperLimit=inf  LowerLimit=1
  T_x : Fcn  Expr=u[1]*cos(u[2])
  T_y : Fcn  Expr=0
  T_z : Fcn  Expr=-u[1]*sin(u[2])
  eta_plr : Outport  VectorParamsAs1DForOutWhenUnconnected=off
  Q : Outport  Port=2
  T : Outport  Port=3  VectorParamsAs1DForOutWhenUnconnected=off
  rpm : Outport  Port=4  VectorParamsAs1DForOutWhenUnconnected=off
  wires:
  Saturation/1 -> Motor/4(rpm0)
  rpm0/1 -> Saturation/1
  "Propeller "/2(T (N)) -> [T]
  dt/1 -> Motor/2(dt)
  Motor/1(rpm) -> rpm/1, Gain4/1, "Propeller "/1(rpm)
  "Propeller "/3(eta_p) -> eta_plr/1
  rho/1 -> [rho]
  "Propeller "/1(P_plr (w)) -> Motor/1(P_shaft), Product/1
  theta_b/1 -> Motor/6(theta_b), "Propeller "/4(theta_b)
  Gain4/1 -> Product/2  "omega"
  T_y/1 -> Mux2/2
  Mux1/1 -> T_z/1, T_x/1, T_y/1
  T_x/1 -> Mux2/1
  i/1 -> [i]
  T_z/1 -> Mux2/3
  Mux2/1 -> T/1
  [T] -> Mux1/1
  Mux4/1 -> Q/1
  [i] -> Mux3/2
  Q_z/1 -> Mux4/3
  Q_x/1 -> Mux4/1
  Mux3/1 -> Q_z/1, Q_x/1, Q_y/1
  Q_y/1 -> Mux4/2
  [Q] -> Mux3/1
  [i] -> Mux1/2
  Product/1 -> Gain2/1
  [V] -> Motor/3(V)
  [V] -> "Propeller "/2(V)
  [rho] -> Motor/5(rho)
  [rho] -> "Propeller "/3(rho)
  Constant/1 -> Manual Switch/1
  V/1 -> [V]
  Gain2/1 -> [Q]

== system eVTOL_PX4_2023b/Subsystem1/Energy & Power/thrust_4 ==
  note: 将推力、扭矩按电机倾转角转化为向量
  note: 求桨的推力、扭矩、功率、效率
  dt : Inport
  V : Inport  Port=2
  rho : Inport  Port=3
  rpm0 : Inport  Port=4
  theta_b : Inport  Port=5
  i : Inport  Port=6
  Constant : Constant  Commented=on  Value=2.5
  Gain4 : Gain  Gain=pi/30
  Manual Switch : ManualSwitch  Commented=on  CurrentSetting=0
  Motor : Subsystem
  Mux1 : Mux  Inputs=2
  Mux2 : Mux  Inputs=3
  Mux3 : Mux  Inputs=2
  Mux4 : Mux  Inputs=3
  Product : Product  Inputs=*/
  "Propeller " : Subsystem
  Q_x : Fcn  Expr=-u[1]*cos(u[2])
  Q_y : Fcn  Expr=0
  Q_z : Fcn  Expr=u[1]*sin(u[2])
  Saturation : Saturate  UpperLimit=inf  LowerLimit=1
  T_x : Fcn  Expr=u[1]*cos(u[2])
  T_y : Fcn  Expr=0
  T_z : Fcn  Expr=-u[1]*sin(u[2])
  eta_plr : Outport  VectorParamsAs1DForOutWhenUnconnected=off
  Q : Outport  Port=2
  T : Outport  Port=3  VectorParamsAs1DForOutWhenUnconnected=off
  rpm : Outport  Port=4  VectorParamsAs1DForOutWhenUnconnected=off
  wires:
  Saturation/1 -> Motor/4(rpm0)
  rpm0/1 -> Saturation/1
  "Propeller "/2(T (N)) -> [T]
  dt/1 -> Motor/2(dt)
  Motor/1(rpm) -> rpm/1, Gain4/1, "Propeller "/1(rpm)
  "Propeller "/3(eta_p) -> eta_plr/1
  rho/1 -> [rho]
  "Propeller "/1(P_plr (w)) -> Motor/1(P_shaft), Product/1
  theta_b/1 -> Motor/6(theta_b), "Propeller "/4(theta_b)
  Gain4/1 -> Product/2  "omega"
  T_y/1 -> Mux2/2
  Mux1/1 -> T_z/1, T_x/1, T_y/1
  T_x/1 -> Mux2/1
  i/1 -> [i]
  T_z/1 -> Mux2/3
  Mux2/1 -> T/1
  [T] -> Mux1/1
  Mux4/1 -> Q/1
  [i] -> Mux3/2
  Q_z/1 -> Mux4/3
  Q_x/1 -> Mux4/1
  Mux3/1 -> Q_z/1, Q_x/1, Q_y/1
  Q_y/1 -> Mux4/2
  [Q] -> Mux3/1
  [i] -> Mux1/2
  [V] -> Motor/3(V)
  [V] -> "Propeller "/2(V)
  [rho] -> Motor/5(rho)
  [rho] -> "Propeller "/3(rho)
  Product/1 -> [Q]
  Constant/1 -> Manual Switch/1
  V/1 -> [V]

== system eVTOL_PX4_2023b/Subsystem1/Energy & Power/thrust_5 ==
  note: 将推力、扭矩按电机倾转角转化为向量
  note: 求桨的推力、扭矩、功率、效率
  dt : Inport
  V : Inport  Port=2
  rho : Inport  Port=3
  rpm0 : Inport  Port=4
  theta_b : Inport  Port=5
  i : Inport  Port=6
  Constant : Constant  Commented=on  Value=2.5
  Gain2 : Gain  Gain=-1
  Gain4 : Gain  Gain=pi/30
  Manual Switch : ManualSwitch  Commented=on  CurrentSetting=0
  Motor : Subsystem
  Mux1 : Mux  Inputs=2
  Mux2 : Mux  Inputs=3
  Mux3 : Mux  Inputs=2
  Mux4 : Mux  Inputs=3
  Product : Product  Inputs=*/
  "Propeller " : Subsystem
  Q_x : Fcn  Expr=-u[1]*cos(u[2])
  Q_y : Fcn  Expr=0
  Q_z : Fcn  Expr=u[1]*sin(u[2])
  Saturation : Saturate  UpperLimit=inf  LowerLimit=1
  T_x : Fcn  Expr=u[1]*cos(u[2])
  T_y : Fcn  Expr=0
  T_z : Fcn  Expr=-u[1]*sin(u[2])
  eta_plr : Outport  VectorParamsAs1DForOutWhenUnconnected=off
  Q : Outport  Port=2
  T : Outport  Port=3  VectorParamsAs1DForOutWhenUnconnected=off
  rpm : Outport  Port=4  VectorParamsAs1DForOutWhenUnconnected=off
  wires:
  Saturation/1 -> Motor/4(rpm0)
  rpm0/1 -> Saturation/1
  "Propeller "/2(T (N)) -> [T]
  dt/1 -> Motor/2(dt)
  Motor/1(rpm) -> rpm/1, Gain4/1, "Propeller "/1(rpm)
  "Propeller "/3(eta_p) -> eta_plr/1
  rho/1 -> [rho]
  "Propeller "/1(P_plr (w)) -> Motor/1(P_shaft), Product/1
  theta_b/1 -> Motor/6(theta_b), "Propeller "/4(theta_b)
  Gain4/1 -> Product/2  "omega"
  T_y/1 -> Mux2/2
  Mux1/1 -> T_z/1, T_x/1, T_y/1
  T_x/1 -> Mux2/1
  i/1 -> [i]
  T_z/1 -> Mux2/3
  Mux2/1 -> T/1
  [T] -> Mux1/1
  Mux4/1 -> Q/1
  [i] -> Mux3/2
  Q_z/1 -> Mux4/3
  Q_x/1 -> Mux4/1
  Mux3/1 -> Q_z/1, Q_x/1, Q_y/1
  Q_y/1 -> Mux4/2
  [Q] -> Mux3/1
  [i] -> Mux1/2
  Product/1 -> Gain2/1
  [V] -> Motor/3(V)
  [V] -> "Propeller "/2(V)
  [rho] -> Motor/5(rho)
  [rho] -> "Propeller "/3(rho)
  Gain2/1 -> [Q]
  Constant/1 -> Manual Switch/1
  V/1 -> [V]

== system eVTOL_PX4_2023b/Subsystem1/Energy & Power/thrust_6 ==
  note: 将推力、扭矩按电机倾转角转化为向量
  note: 求桨的推力、扭矩、功率、效率
  dt : Inport
  V : Inport  Port=2
  rho : Inport  Port=3
  rpm0 : Inport  Port=4
  theta_b : Inport  Port=5
  i : Inport  Port=6
  Constant : Constant  Commented=on  Value=2.5
  Gain4 : Gain  Gain=pi/30
  Manual Switch : ManualSwitch  Commented=on  CurrentSetting=0
  Motor : Subsystem
  Mux1 : Mux  Inputs=2
  Mux2 : Mux  Inputs=3
  Mux3 : Mux  Inputs=2
  Mux4 : Mux  Inputs=3
  Product : Product  Inputs=*/
  "Propeller " : Subsystem
  Q_x : Fcn  Expr=-u[1]*cos(u[2])
  Q_y : Fcn  Expr=0
  Q_z : Fcn  Expr=u[1]*sin(u[2])
  Saturation : Saturate  UpperLimit=inf  LowerLimit=1
  T_x : Fcn  Expr=u[1]*cos(u[2])
  T_y : Fcn  Expr=0
  T_z : Fcn  Expr=-u[1]*sin(u[2])
  eta_plr : Outport  VectorParamsAs1DForOutWhenUnconnected=off
  Q : Outport  Port=2
  T : Outport  Port=3  VectorParamsAs1DForOutWhenUnconnected=off
  rpm : Outport  Port=4  VectorParamsAs1DForOutWhenUnconnected=off
  wires:
  Saturation/1 -> Motor/4(rpm0)
  rpm0/1 -> Saturation/1
  "Propeller "/2(T (N)) -> [T]
  dt/1 -> Motor/2(dt)
  Motor/1(rpm) -> rpm/1, Gain4/1, "Propeller "/1(rpm)
  "Propeller "/3(eta_p) -> eta_plr/1
  rho/1 -> [rho]
  "Propeller "/1(P_plr (w)) -> Motor/1(P_shaft), Product/1
  theta_b/1 -> Motor/6(theta_b), "Propeller "/4(theta_b)
  Gain4/1 -> Product/2  "omega"
  T_y/1 -> Mux2/2
  Mux1/1 -> T_z/1, T_x/1, T_y/1
  T_x/1 -> Mux2/1
  i/1 -> [i]
  T_z/1 -> Mux2/3
  Mux2/1 -> T/1
  [T] -> Mux1/1
  Mux4/1 -> Q/1
  [i] -> Mux3/2
  Q_z/1 -> Mux4/3
  Q_x/1 -> Mux4/1
  Mux3/1 -> Q_z/1, Q_x/1, Q_y/1
  Q_y/1 -> Mux4/2
  [Q] -> Mux3/1
  [i] -> Mux1/2
  [V] -> Motor/3(V)
  [V] -> "Propeller "/2(V)
  [rho] -> Motor/5(rho)
  [rho] -> "Propeller "/3(rho)
  Product/1 -> [Q]
  Constant/1 -> Manual Switch/1
  V/1 -> [V]

== system eVTOL_PX4_2023b/Subsystem1/Energy & Power1/V_prop1 ==
  note: 将速度矢量投影到桨轴
  pqr : Inport
  pos : Inport  Port=2
  i : Inport  Port=3
  Vb : Inport  Port=4
  Cross Product4 : matrix_library/Cross Product
  Display1 : Display
  Display2 : Display
  Display8 : Display
  Sum2 : Sum  Inputs=|++
  v_b to v_prop : Subsystem
  V : Outport
  wires:
  pos/1 -> Cross Product4/2
  pqr/1 -> Cross Product4/1
  Vb/1 -> Display2/1, Sum2/2
  i/1 -> v_b to v_prop/2(i)
  Cross Product4/1 -> Display8/1, Sum2/1
  Sum2/1 -> Display1/1, v_b to v_prop/1(V_body)
  v_b to v_prop/1(V) -> V/1

== system eVTOL_PX4_2023b/Subsystem1/Energy & Power1/V_prop2 ==
  note: 将速度矢量投影到桨轴
  pqr : Inport
  pos : Inport  Port=2
  i : Inport  Port=3
  Vb : Inport  Port=4
  Cross Product4 : matrix_library/Cross Product
  Sum2 : Sum  Inputs=|++
  v_b to v_prop : Subsystem
  V : Outport
  wires:
  pos/1 -> Cross Product4/2
  pqr/1 -> Cross Product4/1
  Vb/1 -> Sum2/2
  i/1 -> v_b to v_prop/2(i)
  Cross Product4/1 -> Sum2/1
  Sum2/1 -> v_b to v_prop/1(V_body)
  v_b to v_prop/1(V) -> V/1

== system eVTOL_PX4_2023b/Subsystem1/Energy & Power1/V_prop3 ==
  note: 将速度矢量投影到桨轴
  pqr : Inport
  pos : Inport  Port=2
  i : Inport  Port=3
  Va : Inport  Port=4
  Cross Product4 : matrix_library/Cross Product
  Sum2 : Sum  Inputs=|++
  v_b to v_prop : Subsystem
  V : Outport
  wires:
  pos/1 -> Cross Product4/2
  pqr/1 -> Cross Product4/1
  Va/1 -> Sum2/2
  i/1 -> v_b to v_prop/2(i)
  Cross Product4/1 -> Sum2/1
  Sum2/1 -> v_b to v_prop/1(V_body)
  v_b to v_prop/1(V) -> V/1

== system eVTOL_PX4_2023b/Subsystem1/Energy & Power1/V_prop4 ==
  note: 将速度矢量投影到桨轴
  pqr : Inport
  pos : Inport  Port=2
  i : Inport  Port=3
  Va : Inport  Port=4
  Cross Product4 : matrix_library/Cross Product
  Sum2 : Sum  Inputs=|++
  v_b to v_prop : Subsystem
  V : Outport
  wires:
  pos/1 -> Cross Product4/2
  pqr/1 -> Cross Product4/1
  Va/1 -> Sum2/2
  i/1 -> v_b to v_prop/2(i)
  Cross Product4/1 -> Sum2/1
  Sum2/1 -> v_b to v_prop/1(V_body)
  v_b to v_prop/1(V) -> V/1

== system eVTOL_PX4_2023b/Subsystem1/Energy & Power1/V_prop5 ==
  note: 将速度矢量投影到桨轴
  pqr : Inport
  pos : Inport  Port=2
  i : Inport  Port=3
  Va : Inport  Port=4
  Cross Product4 : matrix_library/Cross Product
  Sum2 : Sum  Inputs=|++
  v_b to v_prop : Subsystem
  V : Outport
  wires:
  pos/1 -> Cross Product4/2
  pqr/1 -> Cross Product4/1
  Va/1 -> Sum2/2
  i/1 -> v_b to v_prop/2(i)
  Cross Product4/1 -> Sum2/1
  Sum2/1 -> v_b to v_prop/1(V_body)
  v_b to v_prop/1(V) -> V/1

== system eVTOL_PX4_2023b/Subsystem1/Energy & Power1/V_prop6 ==
  note: 将速度矢量投影到桨轴
  pqr : Inport
  pos : Inport  Port=2
  i : Inport  Port=3
  Va : Inport  Port=4
  Cross Product4 : matrix_library/Cross Product
  Sum2 : Sum  Inputs=|++
  v_b to v_prop : Subsystem
  V : Outport
  wires:
  pos/1 -> Cross Product4/2
  pqr/1 -> Cross Product4/1
  Va/1 -> Sum2/2
  i/1 -> v_b to v_prop/2(i)
  Cross Product4/1 -> Sum2/1
  Sum2/1 -> v_b to v_prop/1(V_body)
  v_b to v_prop/1(V) -> V/1

== system eVTOL_PX4_2023b/Subsystem1/Energy & Power1/thrust_1 ==
  note: 将推力、扭矩按电机倾转角转化为向量
  note: 求桨的推力、扭矩、功率、效率
  dt : Inport
  V : Inport  Port=2
  rho : Inport  Port=3
  rpm0 : Inport  Port=4
  rpm_grid : Inport  Port=5
  i : Inport  Port=6
  Constant : Constant  Commented=on  Value=2.5
  Gain2 : Gain  Gain=-1
  Gain4 : Gain  Gain=pi/30
  Manual Switch : ManualSwitch  Commented=on  CurrentSetting=0
  Motor : Subsystem
  Mux1 : Mux  Inputs=2
  Mux2 : Mux  Inputs=3
  Mux3 : Mux  Inputs=2
  Mux4 : Mux  Inputs=3
  Product : Product  Inputs=*/
  "Propeller " : Subsystem
  Q_x : Fcn  Expr=-u[1]*cos(u[2])
  Q_y : Fcn  Expr=0
  Q_z : Fcn  Expr=u[1]*sin(u[2])
  Saturation : Saturate  UpperLimit=inf  LowerLimit=1
  T_x : Fcn  Expr=u[1]*cos(u[2])
  T_y : Fcn  Expr=0
  T_z : Fcn  Expr=-u[1]*sin(u[2])
  eta_plr : Outport  VectorParamsAs1DForOutWhenUnconnected=off
  Q : Outport  Port=2
  T : Outport  Port=3  VectorParamsAs1DForOutWhenUnconnected=off
  rpm : Outport  Port=4  VectorParamsAs1DForOutWhenUnconnected=off
  wires:
  Saturation/1 -> Motor/4(rpm0)
  rpm0/1 -> Saturation/1
  "Propeller "/2(T (N)) -> [T]
  dt/1 -> Motor/2(dt)
  Motor/1(rpm) -> rpm/1, Gain4/1, "Propeller "/1(rpm)
  "Propeller "/3(eta_p) -> eta_plr/1
  rho/1 -> [rho]
  "Propeller "/1(P_plr (w)) -> Motor/1(P_shaft), Product/1
  Gain4/1 -> Product/2  "omega"
  Product/1 -> Gain2/1
  T_y/1 -> Mux2/2
  Mux1/1 -> T_z/1, T_x/1, T_y/1
  T_x/1 -> Mux2/1
  i/1 -> [i]
  T_z/1 -> Mux2/3
  Mux2/1 -> T/1
  [T] -> Mux1/1
  Mux4/1 -> Q/1
  [i] -> Mux3/2
  Q_z/1 -> Mux4/3
  Q_x/1 -> Mux4/1
  Mux3/1 -> Q_z/1, Q_x/1, Q_y/1
  Q_y/1 -> Mux4/2
  [Q] -> Mux3/1
  [i] -> Mux1/2
  Gain2/1 -> [Q]
  [V] -> Motor/3(V)
  [V] -> "Propeller "/2(V)
  [rho] -> Motor/5(rho)
  [rho] -> "Propeller "/3(rho)
  Constant/1 -> Manual Switch/1
  V/1 -> [V]
  rpm_grid/1 -> Motor/6(rpm_grid)

== system eVTOL_PX4_2023b/Subsystem1/Energy & Power1/thrust_2 ==
  note: 将推力、扭矩按电机倾转角转化为向量
  note: 求桨的推力、扭矩、功率、效率
  dt : Inport
  V : Inport  Port=2
  rho : Inport  Port=3
  rpm0 : Inport  Port=4
  rpm_grid : Inport  Port=5
  i : Inport  Port=6
  Constant : Constant  Commented=on  Value=2.5
  Gain4 : Gain  Gain=pi/30
  Manual Switch : ManualSwitch  Commented=on  CurrentSetting=0
  Motor : Subsystem
  Mux1 : Mux  Inputs=2
  Mux2 : Mux  Inputs=3
  Mux3 : Mux  Inputs=2
  Mux4 : Mux  Inputs=3
  Product : Product  Inputs=*/
  "Propeller " : Subsystem
  Q_x : Fcn  Expr=-u[1]*cos(u[2])
  Q_y : Fcn  Expr=0
  Q_z : Fcn  Expr=u[1]*sin(u[2])
  Saturation : Saturate  UpperLimit=inf  LowerLimit=1
  T_x : Fcn  Expr=u[1]*cos(u[2])
  T_y : Fcn  Expr=0
  T_z : Fcn  Expr=-u[1]*sin(u[2])
  eta_plr : Outport  VectorParamsAs1DForOutWhenUnconnected=off
  Q : Outport  Port=2
  T : Outport  Port=3  VectorParamsAs1DForOutWhenUnconnected=off
  rpm : Outport  Port=4  VectorParamsAs1DForOutWhenUnconnected=off
  wires:
  Saturation/1 -> Motor/4(rpm0)
  rpm0/1 -> Saturation/1
  "Propeller "/2(T (N)) -> [T]
  dt/1 -> Motor/2(dt)
  Motor/1(rpm) -> rpm/1, Gain4/1, "Propeller "/1(rpm)
  "Propeller "/3(eta_p) -> eta_plr/1
  rho/1 -> [rho]
  "Propeller "/1(P_plr (w)) -> Motor/1(P_shaft), Product/1
  rpm_grid/1 -> Motor/6(rpm_grid)
  Gain4/1 -> Product/2  "omega"
  T_y/1 -> Mux2/2
  Mux1/1 -> T_z/1, T_x/1, T_y/1
  T_x/1 -> Mux2/1
  i/1 -> [i]
  T_z/1 -> Mux2/3
  Mux2/1 -> T/1
  [T] -> Mux1/1
  Mux4/1 -> Q/1
  [i] -> Mux3/2
  Q_z/1 -> Mux4/3
  Q_x/1 -> Mux4/1
  Mux3/1 -> Q_z/1, Q_x/1, Q_y/1
  Q_y/1 -> Mux4/2
  [Q] -> Mux3/1
  [i] -> Mux1/2
  Product/1 -> [Q]
  [V] -> Motor/3(V)
  [V] -> "Propeller "/2(V)
  [rho] -> Motor/5(rho)
  [rho] -> "Propeller "/3(rho)
  Constant/1 -> Manual Switch/1
  V/1 -> [V]

== system eVTOL_PX4_2023b/Subsystem1/Energy & Power1/thrust_3 ==
  note: 将推力、扭矩按电机倾转角转化为向量
  note: 求桨的推力、扭矩、功率、效率
  dt : Inport
  V : Inport  Port=2
  rho : Inport  Port=3
  rpm0 : Inport  Port=4
  rpm_grid : Inport  Port=5
  i : Inport  Port=6
  Constant : Constant  Commented=on  Value=2.5
  Gain4 : Gain  Gain=pi/30
  Manual Switch : ManualSwitch  Commented=on  CurrentSetting=0
  Motor : Subsystem
  Mux1 : Mux  Inputs=2
  Mux2 : Mux  Inputs=3
  Mux3 : Mux  Inputs=2
  Mux4 : Mux  Inputs=3
  Product : Product  Inputs=*/
  "Propeller " : Subsystem
  Q_x : Fcn  Expr=-u[1]*cos(u[2])
  Q_y : Fcn  Expr=0
  Q_z : Fcn  Expr=u[1]*sin(u[2])
  Saturation : Saturate  UpperLimit=inf  LowerLimit=1
  T_x : Fcn  Expr=u[1]*cos(u[2])
  T_y : Fcn  Expr=0
  T_z : Fcn  Expr=-u[1]*sin(u[2])
  eta_plr : Outport  VectorParamsAs1DForOutWhenUnconnected=off
  Q : Outport  Port=2
  T : Outport  Port=3  VectorParamsAs1DForOutWhenUnconnected=off
  rpm : Outport  Port=4  VectorParamsAs1DForOutWhenUnconnected=off
  wires:
  Saturation/1 -> Motor/4(rpm0)
  rpm0/1 -> Saturation/1
  "Propeller "/2(T (N)) -> [T]
  dt/1 -> Motor/2(dt)
  Motor/1(rpm) -> rpm/1, Gain4/1, "Propeller "/1(rpm)
  "Propeller "/3(eta_p) -> eta_plr/1
  rho/1 -> [rho]
  "Propeller "/1(P_plr (w)) -> Motor/1(P_shaft), Product/1
  rpm_grid/1 -> Motor/6(rpm_grid)
  Gain4/1 -> Product/2  "omega"
  T_y/1 -> Mux2/2
  Mux1/1 -> T_z/1, T_x/1, T_y/1
  T_x/1 -> Mux2/1
  i/1 -> [i]
  T_z/1 -> Mux2/3
  Mux2/1 -> T/1
  [T] -> Mux1/1
  Mux4/1 -> Q/1
  [i] -> Mux3/2
  Q_z/1 -> Mux4/3
  Q_x/1 -> Mux4/1
  Mux3/1 -> Q_z/1, Q_x/1, Q_y/1
  Q_y/1 -> Mux4/2
  [Q] -> Mux3/1
  [i] -> Mux1/2
  Product/1 -> [Q]
  [V] -> Motor/3(V)
  [V] -> "Propeller "/2(V)
  [rho] -> Motor/5(rho)
  [rho] -> "Propeller "/3(rho)
  Constant/1 -> Manual Switch/1
  V/1 -> [V]

== system eVTOL_PX4_2023b/Subsystem1/Energy & Power1/thrust_4 ==
  note: 将推力、扭矩按电机倾转角转化为向量
  note: 求桨的推力、扭矩、功率、效率
  dt : Inport
  V : Inport  Port=2
  rho : Inport  Port=3
  rpm0 : Inport  Port=4
  rpm_grid : Inport  Port=5
  i : Inport  Port=6
  Constant : Constant  Commented=on  Value=2.5
  Gain2 : Gain  Gain=-1
  Gain4 : Gain  Gain=pi/30
  Manual Switch : ManualSwitch  Commented=on  CurrentSetting=0
  Motor : Subsystem
  Mux1 : Mux  Inputs=2
  Mux2 : Mux  Inputs=3
  Mux3 : Mux  Inputs=2
  Mux4 : Mux  Inputs=3
  Product : Product  Inputs=*/
  "Propeller " : Subsystem
  Q_x : Fcn  Expr=-u[1]*cos(u[2])
  Q_y : Fcn  Expr=0
  Q_z : Fcn  Expr=u[1]*sin(u[2])
  Saturation : Saturate  UpperLimit=inf  LowerLimit=1
  T_x : Fcn  Expr=u[1]*cos(u[2])
  T_y : Fcn  Expr=0
  T_z : Fcn  Expr=-u[1]*sin(u[2])
  eta_plr : Outport  VectorParamsAs1DForOutWhenUnconnected=off
  Q : Outport  Port=2
  T : Outport  Port=3  VectorParamsAs1DForOutWhenUnconnected=off
  rpm : Outport  Port=4  VectorParamsAs1DForOutWhenUnconnected=off
  wires:
  Saturation/1 -> Motor/4(rpm0)
  rpm0/1 -> Saturation/1
  "Propeller "/2(T (N)) -> [T]
  dt/1 -> Motor/2(dt)
  Motor/1(rpm) -> rpm/1, Gain4/1, "Propeller "/1(rpm)
  "Propeller "/3(eta_p) -> eta_plr/1
  rho/1 -> [rho]
  "Propeller "/1(P_plr (w)) -> Motor/1(P_shaft), Product/1
  rpm_grid/1 -> Motor/6(rpm_grid)
  Gain4/1 -> Product/2  "omega"
  T_y/1 -> Mux2/2
  Mux1/1 -> T_z/1, T_x/1, T_y/1
  T_x/1 -> Mux2/1
  i/1 -> [i]
  T_z/1 -> Mux2/3
  Mux2/1 -> T/1
  [T] -> Mux1/1
  Mux4/1 -> Q/1
  [i] -> Mux3/2
  Q_z/1 -> Mux4/3
  Q_x/1 -> Mux4/1
  Mux3/1 -> Q_z/1, Q_x/1, Q_y/1
  Q_y/1 -> Mux4/2
  [Q] -> Mux3/1
  [i] -> Mux1/2
  Product/1 -> Gain2/1
  [V] -> Motor/3(V)
  [V] -> "Propeller "/2(V)
  [rho] -> Motor/5(rho)
  [rho] -> "Propeller "/3(rho)
  Gain2/1 -> [Q]
  Constant/1 -> Manual Switch/1
  V/1 -> [V]
